simulink model "Orbit_Calc"  (R2024b)
settings: Solver=VariableStepAuto  StartTime=0.0  StopTime=T  FixedStep=1  RelTol=1e-3
values from neighbouring files (symbols this model uses):
  auto_planet = 1    [Inc_Energies.m]    (also in Temps_Hot_Cold.m)
  jtim = juliandate(2000, 1, 1, 0, 0, tim-tau)    [Inc_Energies.m]    (also in Temps_Hot_Cold.m)
  pat = struct("Faces", patc.Faces, "Vertices", patc.Vertices, "UserData",     patc.UserData)    [Temps_Hot_Cold.m]    (also in VenusUranus_energies.mat = ; geometry.m)
  planet_num = 0    [Inc_Energies.m]    (also in Temps_Hot_Cold.m)
libraries: matrix_library x5
settings Model: Creator=Adam  LastModifiedBy=Adam
settings DataIOCC: OutputOption=SpecifiedOutputTimes  OutputTimes=0:T/steps:T

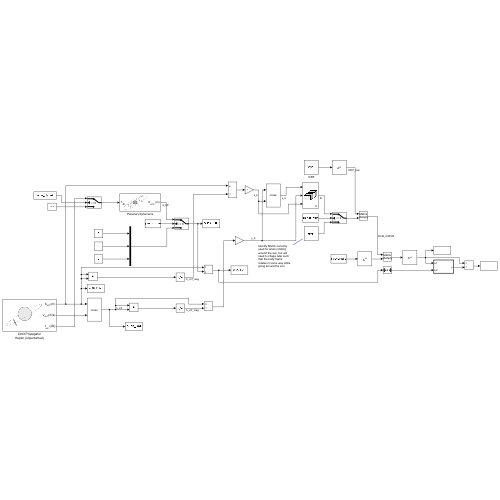
[thumbnail: Simulink's stored preview of the top-level diagram]
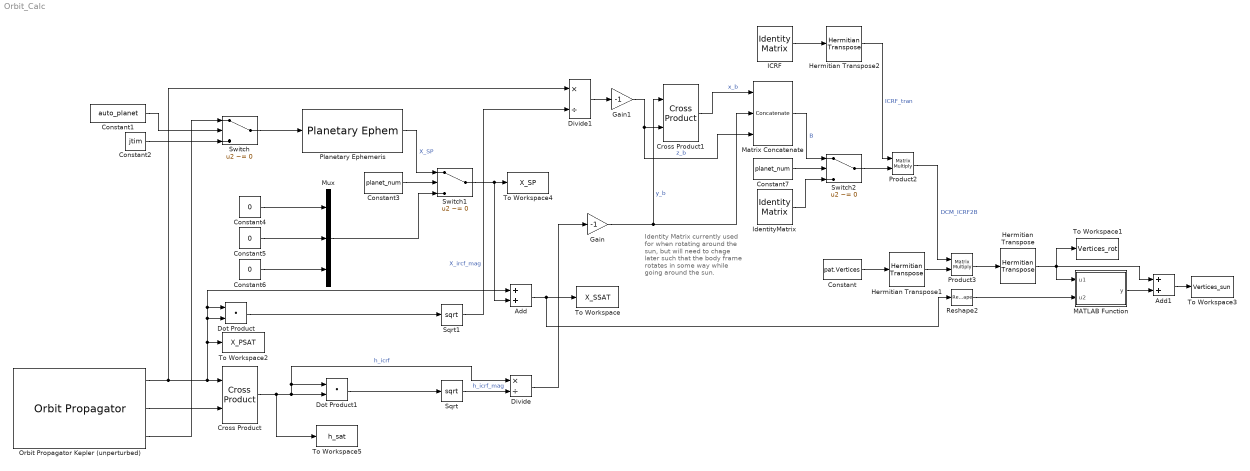
== system Orbit_Calc ==
  note: Identity Matrix currently used for when rotating around the sun, but will need to chage later such that the body frame rotates in some way while going around the sun.
  Add : Sum
  Add1 : Sum
  Constant : Constant  Value=pat.Vertices
  Constant1 : Constant  Value=auto_planet
  Constant2 : Constant  Value=jtim
  Constant3 : Constant  Value=planet_num
  Constant4 : Constant  Value=0
  Constant5 : Constant  Value=0
  Constant6 : Constant  Value=0
  Constant7 : Constant  Value=planet_num
  Cross Product : matrix_library/Cross Product
  Cross Product1 : matrix_library/Cross Product
  Divide : Product  Inputs=*/
  Divide1 : Product  Inputs=*/
  Dot Product : DotProduct  OutDataTypeStr=Inherit: Inherit via internal rule
  Dot Product1 : DotProduct  OutDataTypeStr=Inherit: Inherit via internal rule
  Gain : Gain  Gain=-1
  Gain1 : Gain  Gain=-1
  Hermitian Transpose : matrix_library/Hermitian Transpose
      settings: LibrarySourceBlock=|
      | simulink/Matrix
      | Operations/Hermitian Transpose
  Hermitian Transpose1 : matrix_library/Hermitian Transpose
      settings: LibrarySourceBlock=|
      | simulink/Matrix
      | Operations/Hermitian Transpose
  Hermitian Transpose2 : matrix_library/Hermitian Transpose
      settings: LibrarySourceBlock=|
      | simulink/Matrix
      | Operations/Hermitian Transpose
  ICRF : IdentityMatrix  OutputDimensions=3
  IdentityMatrix : IdentityMatrix  OutputDimensions=3
  MATLAB Function : MATLAB Function  TreatAsAtomicUnit=on
  Matrix Concatenate : Concatenate  NumInputs=3  Mode=Multidimensional array  ConcatenateDimension=2
  Mux : Mux  Inputs=3
  Orbit Propagator Kepler (unperturbed) : OrbitPropagator  startDate=jtim_0  semiMajorAxis=a_sat  eccentricity=e_sat  inclination=i_sat  raan=R_sat  argPeriapsis=w_sat  trueAnomaly=f_sat  argLat=w_sat  inertialPosition=[3649700.0 3308200.0 -4676600.0]  inertialVelocity=[-2750.8 6666.4 2573.4]  fixedPosition=[-4142689.0 -2676864.7 -4669861.6]  fixedVelocity=[1452.7 -6720.7 2568.1]  centralBody=Uranus  customR=3396200  customMu=4.305e13  customJ2=1.0826269e-03  customOmega=4.06125949e-3  includeMoonGravity=off
  Planetary Ephemeris : PlanetaryEphem  units=m,m/s  center=Sun  target=Uranus  outputVelocity=off
  Product2 : Product  Multiplication=Matrix(*)
  Product3 : Product  Multiplication=Matrix(*)
  Reshape2 : Reshape  OutputDimensionality=Row vector (2-D)
  Sqrt : Sqrt
  Sqrt1 : Sqrt
  Switch : Switch  Criteria=u2 ~= 0  SaturateOnIntegerOverflow=off  InputSameDT=off
  Switch1 : Switch  Criteria=u2 ~= 0  SaturateOnIntegerOverflow=off  InputSameDT=off
  Switch2 : Switch  Criteria=u2 ~= 0  SaturateOnIntegerOverflow=off  InputSameDT=off
  To Workspace : ToWorkspace  VariableName=X_SSAT  SampleTime=-1
      settings: Save2DSignal=2-D array (concatenate along first dimension)
  To Workspace1 : ToWorkspace  VariableName=Vertices_rot  SampleTime=-1
  To Workspace2 : ToWorkspace  VariableName=X_PSAT  SampleTime=-1
      settings: Save2DSignal=2-D array (concatenate along first dimension)
  To Workspace3 : ToWorkspace  VariableName=Vertices_sun  SampleTime=-1
  To Workspace4 : ToWorkspace  VariableName=X_SP  SampleTime=-1
      settings: Save2DSignal=2-D array (concatenate along first dimension)
  To Workspace5 : ToWorkspace  VariableName=h_sat  SampleTime=-1
      settings: Save2DSignal=2-D array (concatenate along first dimension)
  wires:
  Constant2/1 -> Switch/3
  Constant1/1 -> Switch/2
  Orbit Propagator Kepler (unperturbed)/1 -> Add/1, Dot Product/1, Dot Product/2, To Workspace2/1, Cross Product/1, Divide1/1
  Constant4/1 -> Mux/1
  Matrix Concatenate/1 -> Switch2/1  "B"
  Orbit Propagator Kepler (unperturbed)/3 -> Switch/1
  Orbit Propagator Kepler (unperturbed)/2 -> Cross Product/2
  Switch/1 -> Planetary Ephemeris/1
  Constant6/1 -> Mux/3
  Constant5/1 -> Mux/2
  Dot Product/1 -> Sqrt1/1
  Cross Product/1 -> To Workspace5/1, Divide/1, Dot Product1/1, Dot Product1/2  "h_icrf"
  Reshape2/1 -> MATLAB Function/2(u2)
  Planetary Ephemeris/1 -> Switch1/1  "X_SP"
  Constant3/1 -> Switch1/2
  Mux/1 -> Switch1/3
  Dot Product1/1 -> Sqrt/1
  Switch1/1 -> To Workspace4/1, Add/2
  Sqrt1/1 -> Divide1/2  "X_ircf_mag"
  Sqrt/1 -> Divide/2  "h_icrf_mag"
  Hermitian Transpose2/1 -> Product2/1  "ICRF_tran"
  Add/1 -> Reshape2/1, To Workspace/1
  Divide/1 -> Gain/1
  Gain/1 -> Matrix Concatenate/2, Cross Product1/1  "y_b"
  Cross Product1/1 -> Matrix Concatenate/1  "x_b"
  Constant7/1 -> Switch2/2
  ICRF/1 -> Hermitian Transpose2/1
  IdentityMatrix/1 -> Switch2/3
  Switch2/1 -> Product2/2
  Constant/1 -> Hermitian Transpose1/1
  Product2/1 -> Product3/1  "DCM_ICRF2B"
  Hermitian Transpose1/1 -> Product3/2
  Product3/1 -> Hermitian Transpose/1
  Hermitian Transpose/1 -> Add1/1, MATLAB Function/1(u1), To Workspace1/1
  MATLAB Function/1(y) -> Add1/2
  Add1/1 -> To Workspace3/1
  Gain1/1 -> Matrix Concatenate/3, Cross Product1/2  "z_b"
  Divide1/1 -> Gain1/1

== matlab function Orbit_Calc/MATLAB Function ==
  data: u1 input; y output; u2 input
function y = repmat_u2(u1, u2)
    le_u1 = size(u1, 1);
    y = repmat(u2, le_u1, 1);
end
